simulink model "example_House_RoomFloorHeating_2"  (R2018b)
settings: Solver=ode45  StartTime=0.0  StopTime=24*3600  RelTol=1e-3  EnableMultiTasking=on
undefined symbols (not defined in the file): path_carnot
libraries: carnot x17
settings Model: SimulationMode=accelerator  Creator=drhf  LastModifiedBy=P41573
settings DataIOCC: LimitDataPoints=on  SaveFormat=Array
settings OptimizationCC: ExpressionDepthLimit=2147483647  LifeSpan=inf
settings DebuggingCC: UnderspecifiedInitializationDetection=Classic  MergeDetectMultiDrivingBlocksExec=none  SolverPrmCheckMsg=warning  StateNameClashWarn=warning  SFUnexpectedBacktrackingDiag=warning  SFNoUnconditionalDefaultTransitionDiag=warning  SFExecutionAtInitializationDiag=none
settings HardwareCC: ProdBitPerPointer=32  ProdBitPerSizeT=32  ProdBitPerPtrDiffT=32  ProdLargestAtomicFloat=None  ProdIntDivRoundTo=Undefined  ProdEndianess=Unspecified  ProdWordSize=32  ProdHWDeviceType=32-bit Generic
settings ModelReferenceCC: PropagateSignalLabelsOutOfModel=off
settings SFSimCC: SimUseLocalCustomCode=off
settings RTWCC: RTWUseLocalCustomCode=off
settings CodeAppCC: StateflowObjectComments=on
settings GRTTargetCC: TargetLangStandard=C89/C90 (ANSI)  GeneratePreprocessorConditionals=Disable all  CombineOutputUpdateFcns=off  GRTInterface=on
settings ConfigComp: CovMetricSettings=dw  CovHtmlReporting=on  CovSaveCumulativeToWorkspaceVar=on  CovSaveSingleToWorkspaceVar=on  CovExternalEMLEnable=off

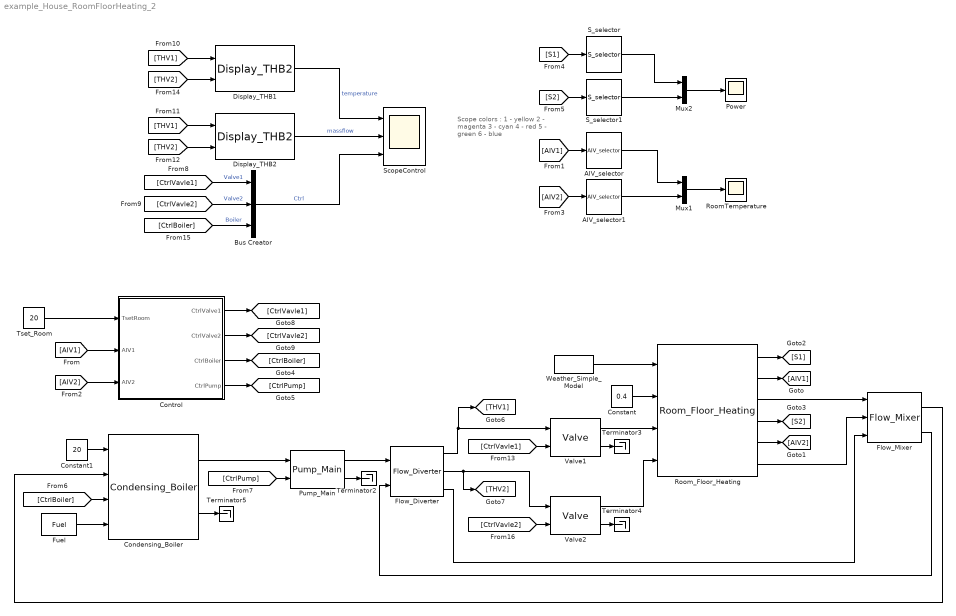
== system example_House_RoomFloorHeating_2 ==
  note: Scope colors :
      | 1 - yellow
      | 2 - magenta
      | 3 - cyan
      | 4 - red
      | 5 - green
      | 6 - blue
  AIV_selector : carnot/Outputs/AIV_selector  e1=off  e2=on  e3=off  e4=off  e5=off  e6=off  e7=off  e8=off  e9=off
      settings: SourceProductName=Carnot
  AIV_selector1 : carnot/Outputs/AIV_selector  e1=off  e2=on  e3=off  e4=off  e5=off  e6=off  e7=off  e8=off  e9=off
      settings: SourceProductName=Carnot
  Bus Creator : BusCreator  Inputs=3
  Condensing_Boiler : carnot/Source/Boiler/Condensing_Boiler  Tini=20  PathName=fullfile(path_carnot('libsl'), 'Source','Boiler','Condensing_Boiler', 'parameter_set')  FileName='CondensingBoiler_10kW.mat'  userPath=off  userParam=off  Pgas=10000  HeatLoss=2.5  Volume=0.0035  whichTforEfficiency=mean of inlet and outlet temperature  TableRelativePower=[0 0.1 1]  TableTemperatures=[10 50 90]  TableData=[1 1 1; 1.08 0.92 0.85; 1.06 0.9 0.83]  ElectricPower=[0 50 200]  relQdotMin=0.1  dplin=10  dpqua=100  nodes=3
      settings: SourceProductName=Carnot
  Constant : Constant  Value=0.4
  Constant1 : Constant  Value=20
  Control : Subsystem
  Display_THB1 : carnot/Outputs/Display_THB2  t=on  m=off  p=off  id=off  mix=off  d=off
      settings: SourceProductName=Carnot
  Display_THB2 : carnot/Outputs/Display_THB2  t=off  m=on  p=off  id=off  mix=off  d=off
      settings: SourceProductName=Carnot
  Flow_Diverter : carnot/Hydraulics/Flow_Diverter
      settings: SourceProductName=Carnot
  Flow_Mixer : carnot/Hydraulics/Flow_Mixer
      settings: SourceProductName=Carnot
  Fuel : carnot/Source/Energy/Fuel  Temperature=20  Pressure=101300  PathName=fullfile(path_carnot('libsl'), 'Source', 'Energy', 'Fuel', 'parameter_set')  FileName='DefaultFuel_Gas.mat'  userPath=off  userParam=off  ft=1  stoichAir=3.5  combustion_enthalpy=[51400000 56900000]  Tcondensation=[45 25]  massfraction=[0.33 0.67 0 0 0 0]  price=1
      settings: SourceProductName=Carnot
  Mux1 : Mux  Inputs=2
  Mux2 : Mux  Inputs=2
  Power : Scope
  Pump_Main : carnot/Hydraulics/Pump_Main  Tini=20  p0=3e5  IDpreset=pressure drop  fluid=Water  mix=0  mix2=0  mix3=0  t1=1  PathName=fullfile(path_carnot('libsl'), 'Hydraulics', 'Pump_Main', 'parameter_set')  FileName='Pump6m.mat'  userPath=off  userParam=off  a0=60000  a1=-43200  a2=0  dia=0.025  UA=1  mcp=4182  e0=50  e1=28.8  e2=-10.368
      settings: SourceProductName=Carnot
  RoomTemperature : Scope
  Room_Floor_Heating : carnot/Load/Houses/Room_Floor_Heating  t0=21  temp_neighbour=20
      settings: SourceProductName=Carnot
  S_selector : carnot/Outputs/S_selector  e1=off  e2=off  e3=off  e4=off  e5=off  e6=off  e7=on  e8=on  e9=off  e10=off  e11=off  e12=off  e13=off
      settings: SourceProductName=Carnot
  S_selector1 : carnot/Outputs/S_selector  e1=off  e2=off  e3=off  e4=off  e5=off  e6=off  e7=on  e8=on  e9=off  e10=off  e11=off  e12=off  e13=off
      settings: SourceProductName=Carnot
  ScopeControl : Scope  NumInputPorts=3
  Terminator{2..5} (4 alike) : Terminator
  Tset_Room : Constant  Value=20
  Valve1 : carnot/Hydraulics/Valve  vtyp=linear  psi_0=0.04  kvs=0.2*3600/1000  dt_V=30
      settings: SourceProductName=Carnot
  Valve2 : carnot/Hydraulics/Valve  vtyp=linear  psi_0=0.04  kvs=0.2*3600/1000  dt_V=30
      settings: SourceProductName=Carnot
  Weather_Simple_Model : carnot/Weather/Weather_Simple_Model  Ibn=900  Idg=100  tamb=5  deltaTsky=-6  rh=50  precip="10e-3/24/3600           % 10 mm in 24 h"  cloud=0.125  p=1013e2  vw=1  wdir=270  lat=60  colangle=0  colazi=0  colrot=0
      settings: SourceProductName=Carnot
  wires:
  Weather_Simple_Model/1 -> Room_Floor_Heating/1
  Constant/1 -> Room_Floor_Heating/2
  Valve1/2 -> Terminator3/1
  Flow_Diverter/1 -> [THV1], Valve1/1
  Flow_Mixer/1 -> Condensing_Boiler/2
  Display_THB2/1 -> ScopeControl/2  "massflow"
  Flow_Diverter/3 -> Flow_Mixer/3
  Bus Creator/1 -> ScopeControl/3  "Ctrl"
  Flow_Diverter/2 -> [THV2], Valve2/1
  Flow_Mixer/2 -> Flow_Diverter/2
  Pump_Main/2 -> Terminator2/1
  Valve2/2 -> Terminator4/1
  Pump_Main/1 -> Flow_Diverter/1
  Condensing_Boiler/1 -> Pump_Main/1
  Condensing_Boiler/2 -> Terminator5/1
  Constant1/1 -> Condensing_Boiler/1
  Fuel/1 -> Condensing_Boiler/4
  Mux2/1 -> Power/1
  S_selector/1 -> Mux2/1
  AIV_selector1/1 -> Mux1/2
  AIV_selector/1 -> Mux1/1
  S_selector1/1 -> Mux2/2
  Mux1/1 -> RoomTemperature/1
  Valve1/1 -> Room_Floor_Heating/3
  Valve2/1 -> Room_Floor_Heating/4
  Room_Floor_Heating/3 -> Flow_Mixer/1
  Room_Floor_Heating/6 -> Flow_Mixer/2
  Room_Floor_Heating/2 -> [AIV1]
  Room_Floor_Heating/5 -> [AIV2]
  [AIV1] -> AIV_selector/1
  [AIV2] -> AIV_selector1/1
  Room_Floor_Heating/1 -> [S1]
  Room_Floor_Heating/4 -> [S2]
  [S1] -> S_selector/1
  [S2] -> S_selector1/1
  [CtrlBoiler] -> Condensing_Boiler/3
  [CtrlPump] -> Pump_Main/2
  [CtrlVavle1] -> Valve1/2
  [CtrlVavle2] -> Valve2/2
  Tset_Room/1 -> Control/1(TsetRoom)
  [AIV1] -> Control/2(AIV1)
  [AIV2] -> Control/3(AIV2)
  Control/1(CtrlValve1) -> [CtrlVavle1]
  Control/2(CtrlValve2) -> [CtrlVavle2]
  Control/3(CtrlBoiler) -> [CtrlBoiler]
  [CtrlVavle1] -> Bus Creator/1  "Valve1"
  [CtrlVavle2] -> Bus Creator/2  "Valve2"
  [THV1] -> Display_THB2/1
  [THV2] -> Display_THB2/2
  [THV2] -> Display_THB1/2
  [THV1] -> Display_THB1/1
  Display_THB1/1 -> ScopeControl/1  "temperature"
  [CtrlBoiler] -> Bus Creator/3  "Boiler"
  Control/4(CtrlPump) -> [CtrlPump]

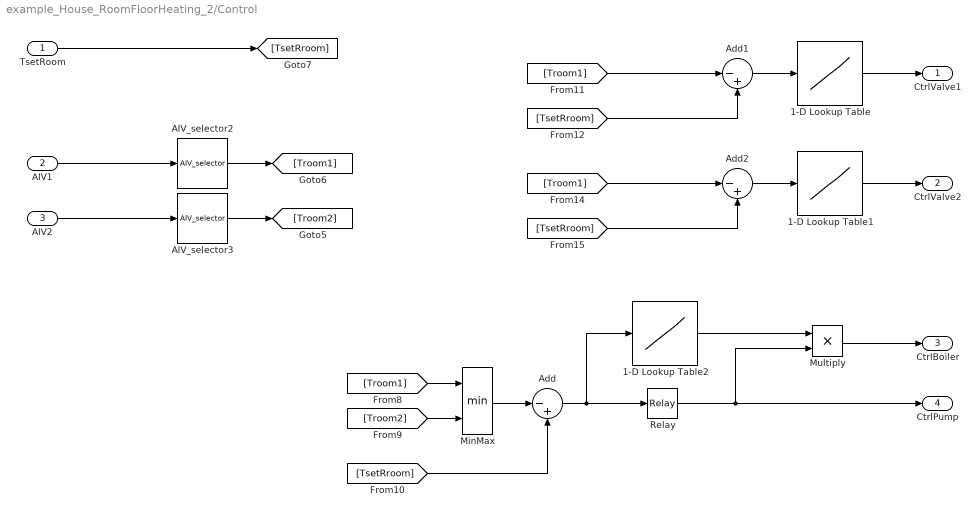
== system example_House_RoomFloorHeating_2/Control ==
  TsetRoom : Inport
  AIV1 : Inport  Port=2
  AIV2 : Inport  Port=3
  1-D Lookup Table : Lookup_n-D  NumberOfTableDimensions=1  BreakpointsForDimension1=[-2 2]  Table=[0 1]  ExtrapMethod=Clip  UseLastTableValue=on  InternalRulePriority=Speed  RndMeth=Simplest  InputSameDT=on
  1-D Lookup Table1 : Lookup_n-D  NumberOfTableDimensions=1  BreakpointsForDimension1=[-2 2]  Table=[0 1]  ExtrapMethod=Clip  UseLastTableValue=on  InternalRulePriority=Speed  RndMeth=Simplest  InputSameDT=on
  1-D Lookup Table2 : Lookup_n-D  NumberOfTableDimensions=1  BreakpointsForDimension1=[-2 2]  Table=[0.1 1]  ExtrapMethod=Clip  UseLastTableValue=on  InternalRulePriority=Speed  RndMeth=Simplest  InputSameDT=on
  AIV_selector2 : carnot/Outputs/AIV_selector  e1=off  e2=on  e3=off  e4=off  e5=off  e6=off  e7=off  e8=off  e9=off
      settings: SourceProductName=Carnot
  AIV_selector3 : carnot/Outputs/AIV_selector  e1=off  e2=on  e3=off  e4=off  e5=off  e6=off  e7=off  e8=off  e9=off
      settings: SourceProductName=Carnot
  Add : Sum  Inputs=|-+
  Add1 : Sum  Inputs=|-+
  Add2 : Sum  Inputs=|-+
  MinMax : MinMax  Inputs=2
  Multiply : Product
  Relay : Relay  OnSwitchValue=1  OffSwitchValue=-1
  CtrlValve1 : Outport
  CtrlValve2 : Outport  Port=2
  CtrlBoiler : Outport  Port=3
  CtrlPump : Outport  Port=4
  wires:
  [Troom2] -> MinMax/2
  Add2/1 -> 1-D Lookup Table1/1
  MinMax/1 -> Add/1
  AIV2/1 -> AIV_selector3/1
  Add/1 -> Relay/1, 1-D Lookup Table2/1
  [TsetRroom] -> Add1/2
  Add1/1 -> 1-D Lookup Table/1
  [Troom1] -> MinMax/1
  Relay/1 -> Multiply/2, CtrlPump/1
  AIV_selector2/1 -> [Troom1]
  AIV1/1 -> AIV_selector2/1
  [Troom1] -> Add2/1
  1-D Lookup Table1/1 -> CtrlValve2/1
  [TsetRroom] -> Add2/2
  [Troom1] -> Add1/1
  [TsetRroom] -> Add/2
  AIV_selector3/1 -> [Troom2]
  1-D Lookup Table/1 -> CtrlValve1/1
  TsetRoom/1 -> [TsetRroom]
  1-D Lookup Table2/1 -> Multiply/1
  Multiply/1 -> CtrlBoiler/1
